simulink model "DoubleInvertedPendulum"  (R2023b)
settings: Solver=ode45  StartTime=0.0  StopTime=10.0  RelTol=1e-3  EnableMultiTasking=on
values from neighbouring files (symbols this model uses):
  b = 0.1    [Doble_Pendulo.m]
  g = 9.8    [Doble_Pendulo.m]
  l1 = 0.5    [Doble_Pendulo.m]
  l2 = 0.5    [Doble_Pendulo.m]
  m0 = 1    [Doble_Pendulo.m]
  m1 = 0.4    [Doble_Pendulo.m]
  m2 = 0.5    [Doble_Pendulo.m]
settings Model: Creator=hamada  LastModifiedBy=Usuario
settings SolverCC: AlgebraicLoopSolver=TrustRegion
settings DataIOCC: LimitDataPoints=on  SaveFormat=Array  ReturnWorkspaceOutputs=off
settings OptimizationCC: LifeSpan=inf
settings DebuggingCC: UnconnectedInputMsg=warning  UnconnectedOutputMsg=warning  UnconnectedLineMsg=warning  SFUnexpectedBacktrackingDiag=warning  SFNoUnconditionalDefaultTransitionDiag=warning  SFExecutionAtInitializationDiag=none  ArithmeticOperatorsInVariantConditions=warning
settings HardwareCC: ProdBitPerPointer=32  ProdBitPerSizeT=32  ProdBitPerPtrDiffT=32  ProdLargestAtomicFloat=None  ProdIntDivRoundTo=Undefined  ProdEndianess=Unspecified  ProdWordSize=32  ProdHWDeviceType=32-bit Generic
settings ModelReferenceCC: ModelReferenceMinAlgLoopOccurrences=on  PropagateSignalLabelsOutOfModel=off
settings SFSimCC: SimUseLocalCustomCode=off  CustomCodeUndefinedFunction=UseInterfaceOnly
settings RTWCC: RTWUseLocalCustomCode=off
settings CodeAppCC: StateflowObjectComments=on
settings GRTTargetCC: TargetLangStandard=C89/C90 (ANSI)
settings ConfigComp: CovMetricSettings=dw  CovSaveCumulativeToWorkspaceVar=on  CovSaveSingleToWorkspaceVar=on  CovExternalEMLEnable=off

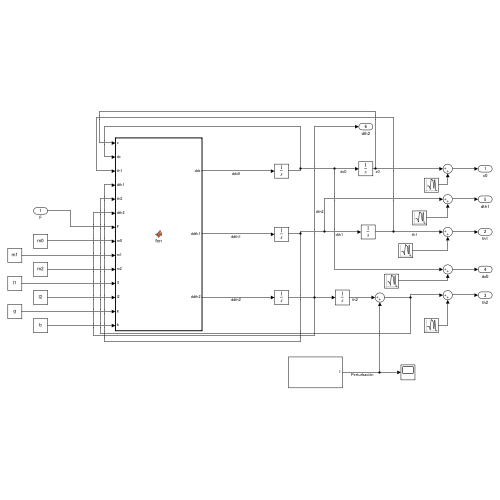
[thumbnail: Simulink's stored preview of the top-level diagram]
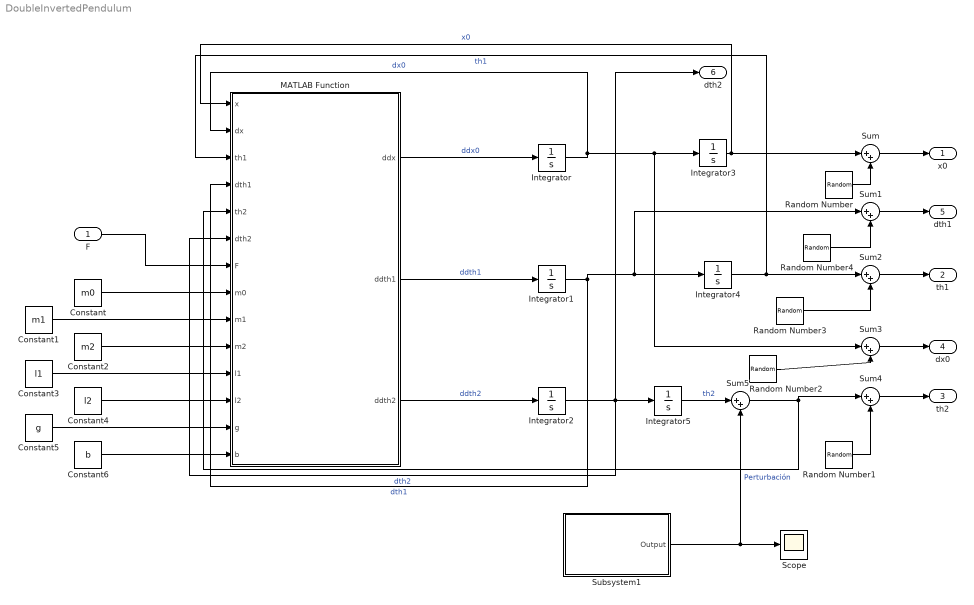
== system DoubleInvertedPendulum ==
  F : Inport
  Constant : Constant  Value=m0
  Constant1 : Constant  Value=m1
  Constant2 : Constant  Value=m2
  Constant3 : Constant  Value=l1
  Constant4 : Constant  Value=l2
  Constant5 : Constant  Value=g
  Constant6 : Constant  Value=b
  Integrator{,1..3} (4 alike) : Integrator
  Integrator4 : Integrator  InitialCondition=0.2
  Integrator5 : Integrator  InitialCondition=-0.2
  MATLAB Function : MATLAB Function  TreatAsAtomicUnit=on
  Random Number : RandomNumber  Variance=0.0001  Seed=10  SampleTime=0.003
  Random Number1 : RandomNumber  Variance=0.00009  Seed=45  SampleTime=0.0015
  Random Number2 : RandomNumber  Variance=0.00002  Seed=111  SampleTime=0.02
  Random Number3 : RandomNumber  Variance=0.0001  Seed=89  SampleTime=0.01
  Random Number4 : RandomNumber  Variance=0.00005  SampleTime=0.004
  Scope : Scope
  Subsystem1 : Subsystem
  Sum{,1..5} (6 alike) : Sum  Inputs=|++
  x0 : Outport
  th1 : Outport  Port=2
  th2 : Outport  Port=3
  dx0 : Outport  Port=4
  dth1 : Outport  Port=5
  dth2 : Outport  Port=6
  wires:
  Integrator5/1 -> Sum5/1  "th2"
  Integrator1/1 -> MATLAB Function/4(dth1), Sum1/1, Integrator4/1  "dth1"
  Integrator3/1 -> MATLAB Function/1(x), Sum/1  "x0"
  Integrator4/1 -> Sum2/1, MATLAB Function/3(th1)  "th1"
  Integrator/1 -> MATLAB Function/2(dx), Sum3/1, Integrator3/1  "dx0"
  Integrator2/1 -> MATLAB Function/6(dth2), Integrator5/1, dth2/1  "dth2"
  MATLAB Function/3(ddth2) -> Integrator2/1  "ddth2"
  MATLAB Function/2(ddth1) -> Integrator1/1  "ddth1"
  MATLAB Function/1(ddx) -> Integrator/1  "ddx0"
  F/1 -> MATLAB Function/7(F)
  Constant/1 -> MATLAB Function/8(m0)
  Constant1/1 -> MATLAB Function/9(m1)
  Constant2/1 -> MATLAB Function/10(m2)
  Constant3/1 -> MATLAB Function/11(l1)
  Constant4/1 -> MATLAB Function/12(l2)
  Constant5/1 -> MATLAB Function/13(g)
  Constant6/1 -> MATLAB Function/14(b)
  Sum/1 -> x0/1
  Sum1/1 -> dth1/1
  Sum2/1 -> th1/1
  Sum3/1 -> dx0/1
  Sum4/1 -> th2/1
  Random Number3/1 -> Sum2/2
  Random Number2/1 -> Sum3/2
  Random Number1/1 -> Sum4/2
  Random Number/1 -> Sum/2
  Random Number4/1 -> Sum1/2
  Sum5/1 -> MATLAB Function/5(th2), Sum4/1
  Subsystem1/1(Output) -> Sum5/2, Scope/1  "Perturbación"

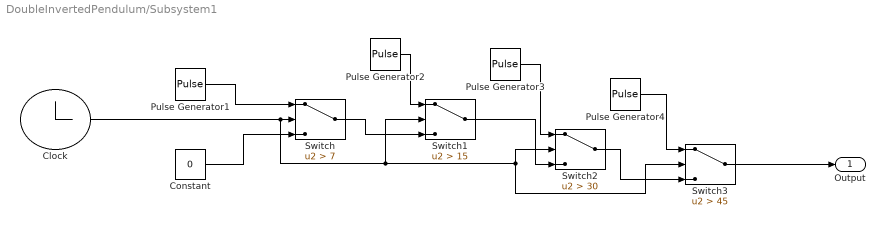
== system DoubleInvertedPendulum/Subsystem1 ==
  Clock : Clock
  Constant : Constant  Value=0
  Pulse Generator1 : DiscretePulseGenerator  PulseType=Time based  Amplitude=0.1  Period=10  PulseWidth=3  PhaseDelay=8
  Pulse Generator2 : DiscretePulseGenerator  PulseType=Time based  Amplitude=0.2  Period=10  PulseWidth=2  PhaseDelay=14
  Pulse Generator3 : DiscretePulseGenerator  PulseType=Time based  Amplitude=0.25  Period=10  PulseWidth=2  PhaseDelay=29
  Pulse Generator4 : DiscretePulseGenerator  PulseType=Time based  Amplitude=0.3  Period=10  PulseWidth=2  PhaseDelay=44
  Switch : Switch  Criteria=u2 > Threshold  Threshold=7  SaturateOnIntegerOverflow=off  InputSameDT=off
  Switch1 : Switch  Criteria=u2 > Threshold  Threshold=15  SaturateOnIntegerOverflow=off  InputSameDT=off
  Switch2 : Switch  Criteria=u2 > Threshold  Threshold=30  SaturateOnIntegerOverflow=off  InputSameDT=off
  Switch3 : Switch  Criteria=u2 > Threshold  Threshold=45  SaturateOnIntegerOverflow=off  InputSameDT=off
  Output : Outport
  wires:
  Pulse Generator1/1 -> Switch/1
  Switch/1 -> Switch1/3
  Switch1/1 -> Switch2/3
  Pulse Generator3/1 -> Switch2/1
  Pulse Generator2/1 -> Switch1/1
  Pulse Generator4/1 -> Switch3/1
  Switch2/1 -> Switch3/3
  Clock/1 -> Switch3/2, Switch2/2, Switch1/2, Switch/2
  Switch3/1 -> Output/1
  Constant/1 -> Switch/3

== matlab function DoubleInvertedPendulum/MATLAB Function ==
  data: ddx output double size=1; ddth1 output double size=1; ddth2 output double size=1; x input; dx input; th1 input; dth1 input; th2 input; dth2 input; F input; m0 input; m1 input; m2 input; l1 input; l2 input; g input; b input
function [ddx,ddth1,ddth2] = fcn(x, dx, th1, dth1,th2, dth2, F, m0, m1, m2, l1, l2, g, b)
    
    % M = [m0+m1+m2 (m1+m2)*l1*cos(th1) (l2*m2*cos(th2));
    %     (m1+m2)*l1*cos(th1) (m1+m2)*l1^2 m2*l1*l2*cos(th1-th2);
    %     m2*l2*cos(th2) m2*l1*l2*cos(th1-th2) m2*l2^2];
    % 
    % f= [l1*(m1+m2)*dth1^2*sin(th1)+m2*l2*dth2^2*sin(th2) - dx*b + F;
    %     -l1*l2*m2*dth2^2*sin(th1-th2)+g*(m1+m2)*l1*sin(th1);
    %     l1*l2*m2*dth1^2*sin(th1-th2)+g*l2*m2*sin(th2)];
    % 
    % x_1=inv(M)*f;
     
    ddx=((l1*l2*m2*sin(th1 - th2)*dth1^2 + g*l2*m2*sin(th2))*(m1*cos(th2) + m2*cos(th2) - m1*cos(th1 - th2)*cos(th1) - m2*cos(th1 - th2)*cos(th1)))/(l2*m2^2*cos(th1 - th2)^2 - l2*m2^2 - l2*m1^2 - l2*m0*m1 - l2*m0*m2 - 2*l2*m1*m2 + l2*m1^2*cos(th1)^2 + l2*m2^2*cos(th1)^2 + l2*m2^2*cos(th2)^2 + l2*m0*m2*cos(th1 - th2)^2 + l2*m1*m2*cos(th1 - th2)^2 + 2*l2*m1*m2*cos(th1)^2 + l2*m1*m2*cos(th2)^2 - 2*l2*m2^2*cos(th1 - th2)*cos(th1)*cos(th2) - 2*l2*m1*m2*cos(th1 - th2)*cos(th1)*cos(th2)) - ((- m2*cos(th1 - th2)^2 + m1 + m2)*(l1*sin(th1)*(m1 + m2)*dth1^2 + l2*m2*sin(th2)*dth2^2 + F - b*dx))/(m1^2*cos(th1)^2 - m0*m2 - 2*m1*m2 - m0*m1 + m2^2*cos(th1)^2 + m2^2*cos(th2)^2 + m2^2*cos(th1 - th2)^2 - m1^2 - m2^2 + 2*m1*m2*cos(th1)^2 + m1*m2*cos(th2)^2 + m0*m2*cos(th1 - th2)^2 + m1*m2*cos(th1 - th2)^2 - 2*m2^2*cos(th1 - th2)*cos(th1)*cos(th2) - 2*m1*m2*cos(th1 - th2)*cos(th1)*cos(th2)) + ((- l1*l2*m2*sin(th1 - th2)*dth2^2 + g*l1*sin(th1)*(m1 + m2))*(m1*cos(th1) + m2*cos(th1) - m2*cos(th1 - th2)*cos(th2)))/(l1*m2^2*cos(th1 - th2)^2 - l1*m2^2 - l1*m1^2 - l1*m0*m1 - l1*m0*m2 - 2*l1*m1*m2 + l1*m1^2*cos(th1)^2 + l1*m2^2*cos(th1)^2 + l1*m2^2*cos(th2)^2 + l1*m0*m2*cos(th1 - th2)^2 + l1*m1*m2*cos(th1 - th2)^2 + 2*l1*m1*m2*cos(th1)^2 + l1*m1*m2*cos(th2)^2 - 2*l1*m2^2*cos(th1 - th2)*cos(th1)*cos(th2) - 2*l1*m1*m2*cos(th1 - th2)*cos(th1)*cos(th2));
    ddth1=((l1*l2*m2*sin(th1 - th2)*dth1^2 + g*l2*m2*sin(th2))*(m0*cos(th1 - th2) + m1*cos(th1 - th2) + m2*cos(th1 - th2) - m1*cos(th1)*cos(th2) - m2*cos(th1)*cos(th2)))/(l1*l2*m1^2*cos(th1)^2 - l1*l2*m2^2 - l1*l2*m0*m1 - l1*l2*m0*m2 - 2*l1*l2*m1*m2 - l1*l2*m1^2 + l1*l2*m2^2*cos(th1)^2 + l1*l2*m2^2*cos(th2)^2 + l1*l2*m2^2*cos(th1 - th2)^2 + 2*l1*l2*m1*m2*cos(th1)^2 + l1*l2*m1*m2*cos(th2)^2 + l1*l2*m0*m2*cos(th1 - th2)^2 + l1*l2*m1*m2*cos(th1 - th2)^2 - 2*l1*l2*m2^2*cos(th1 - th2)*cos(th1)*cos(th2) - 2*l1*l2*m1*m2*cos(th1 - th2)*cos(th1)*cos(th2)) - ((- l1*l2*m2*sin(th1 - th2)*dth2^2 + g*l1*sin(th1)*(m1 + m2))*(- m2*cos(th2)^2 + m0 + m1 + m2))/(l1^2*m1^2*cos(th1)^2 - l1^2*m2^2 - l1^2*m0*m1 - l1^2*m0*m2 - 2*l1^2*m1*m2 - l1^2*m1^2 + l1^2*m2^2*cos(th1)^2 + l1^2*m2^2*cos(th2)^2 + l1^2*m2^2*cos(th1 - th2)^2 + 2*l1^2*m1*m2*cos(th1)^2 + l1^2*m1*m2*cos(th2)^2 + l1^2*m0*m2*cos(th1 - th2)^2 + l1^2*m1*m2*cos(th1 - th2)^2 - 2*l1^2*m2^2*cos(th1 - th2)*cos(th1)*cos(th2) - 2*l1^2*m1*m2*cos(th1 - th2)*cos(th1)*cos(th2)) + ((m1*cos(th1) + m2*cos(th1) - m2*cos(th1 - th2)*cos(th2))*(l1*sin(th1)*(m1 + m2)*dth1^2 + l2*m2*sin(th2)*dth2^2 + F - b*dx))/(l1*m2^2*cos(th1 - th2)^2 - l1*m2^2 - l1*m1^2 - l1*m0*m1 - l1*m0*m2 - 2*l1*m1*m2 + l1*m1^2*cos(th1)^2 + l1*m2^2*cos(th1)^2 + l1*m2^2*cos(th2)^2 + l1*m0*m2*cos(th1 - th2)^2 + l1*m1*m2*cos(th1 - th2)^2 + 2*l1*m1*m2*cos(th1)^2 + l1*m1*m2*cos(th2)^2 - 2*l1*m2^2*cos(th1 - th2)*cos(th1)*cos(th2) - 2*l1*m1*m2*cos(th1 - th2)*cos(th1)*cos(th2));
    ddth2=((m1*cos(th2) + m2*cos(th2) - m1*cos(th1 - th2)*cos(th1) - m2*cos(th1 - th2)*cos(th1))*(l1*sin(th1)*(m1 + m2)*dth1^2 + l2*m2*sin(th2)*dth2^2 + F - b*dx))/(l2*m2^2*cos(th1 - th2)^2 - l2*m2^2 - l2*m1^2 - l2*m0*m1 - l2*m0*m2 - 2*l2*m1*m2 + l2*m1^2*cos(th1)^2 + l2*m2^2*cos(th1)^2 + l2*m2^2*cos(th2)^2 + l2*m0*m2*cos(th1 - th2)^2 + l2*m1*m2*cos(th1 - th2)^2 + 2*l2*m1*m2*cos(th1)^2 + l2*m1*m2*cos(th2)^2 - 2*l2*m2^2*cos(th1 - th2)*cos(th1)*cos(th2) - 2*l2*m1*m2*cos(th1 - th2)*cos(th1)*cos(th2)) + ((- l1*l2*m2*sin(th1 - th2)*dth2^2 + g*l1*sin(th1)*(m1 + m2))*(m0*cos(th1 - th2) + m1*cos(th1 - th2) + m2*cos(th1 - th2) - m1*cos(th1)*cos(th2) - m2*cos(th1)*cos(th2)))/(l1*l2*m1^2*cos(th1)^2 - l1*l2*m2^2 - l1*l2*m0*m1 - l1*l2*m0*m2 - 2*l1*l2*m1*m2 - l1*l2*m1^2 + l1*l2*m2^2*cos(th1)^2 + l1*l2*m2^2*cos(th2)^2 + l1*l2*m2^2*cos(th1 - th2)^2 + 2*l1*l2*m1*m2*cos(th1)^2 + l1*l2*m1*m2*cos(th2)^2 + l1*l2*m0*m2*cos(th1 - th2)^2 + l1*l2*m1*m2*cos(th1 - th2)^2 - 2*l1*l2*m2^2*cos(th1 - th2)*cos(th1)*cos(th2) - 2*l1*l2*m1*m2*cos(th1 - th2)*cos(th1)*cos(th2)) - ((l1*l2*m2*sin(th1 - th2)*dth1^2 + g*l2*m2*sin(th2))*(m0*m1 + m0*m2 + 2*m1*m2 - m1^2*cos(th1)^2 - m2^2*cos(th1)^2 + m1^2 + m2^2 - 2*m1*m2*cos(th1)^2))/(l2^2*m2^3*cos(th1)^2 - l2^2*m2^3 + l2^2*m2^3*cos(th2)^2 + l2^2*m2^3*cos(th1 - th2)^2 - l2^2*m0*m2^2 - 2*l2^2*m1*m2^2 - l2^2*m1^2*m2 - l2^2*m0*m1*m2 + 2*l2^2*m1*m2^2*cos(th1)^2 + l2^2*m1^2*m2*cos(th1)^2 + l2^2*m1*m2^2*cos(th2)^2 + l2^2*m0*m2^2*cos(th1 - th2)^2 + l2^2*m1*m2^2*cos(th1 - th2)^2 - 2*l2^2*m2^3*cos(th1 - th2)*cos(th1)*cos(th2) - 2*l2^2*m1*m2^2*cos(th1 - th2)*cos(th1)*cos(th2));

end
